simulink model "fmincon_in_simulink"  (R2022a)
settings: Solver=VariableStepAuto  StartTime=0.0  StopTime=10.0  RelTol=1e-3
libraries: slpidlib x8
settings Model: Creator=luca9  LastModifiedBy=luca9

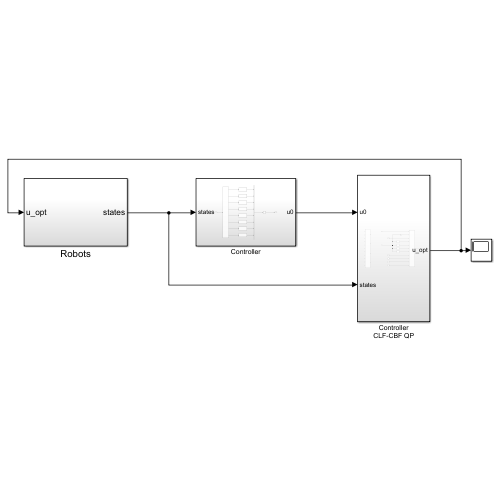
[thumbnail: Simulink's stored preview of the top-level diagram]
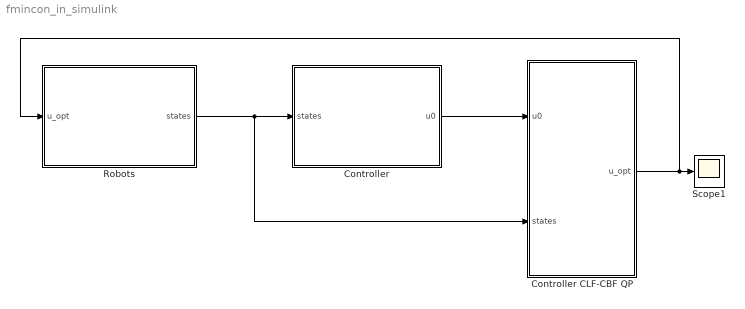
== system fmincon_in_simulink ==
  Controller : Subsystem
  Controller CLF-CBF QP : Subsystem
  Robots : Subsystem
  Scope1 : Scope
  wires:
  Controller CLF-CBF QP/1(u_opt) -> Robots/1(u_opt), Scope1/1
  Robots/1(states) -> Controller/1(states), Controller CLF-CBF QP/2(states)
  Controller/1(u0) -> Controller CLF-CBF QP/1(u0)

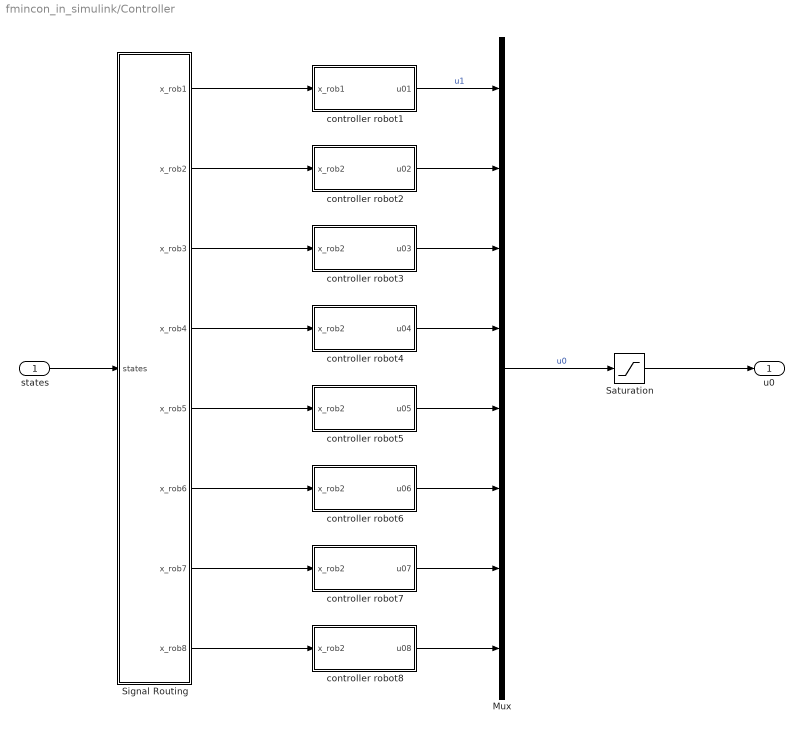
== system fmincon_in_simulink/Controller ==
  states : Inport
  Mux : Mux  Inputs=8
  Saturation : Saturate  UpperLimit=10  LowerLimit=-10
  Signal Routing : MATLAB Function  TreatAsAtomicUnit=on
  controller robot1 : Subsystem
  controller robot2 : Subsystem
  controller robot3 : Subsystem
  controller robot4 : Subsystem
  controller robot5 : Subsystem
  controller robot6 : Subsystem
  controller robot7 : Subsystem
  controller robot8 : Subsystem
  u0 : Outport
  wires:
  states/1 -> Signal Routing/1(states)
  Signal Routing/1(x_rob1) -> controller robot1/1(x_rob1)
  Signal Routing/2(x_rob2) -> controller robot2/1(x_rob2)
  Signal Routing/3(x_rob3) -> controller robot3/1(x_rob2)
  Signal Routing/4(x_rob4) -> controller robot4/1(x_rob2)
  Signal Routing/5(x_rob5) -> controller robot5/1(x_rob2)
  Signal Routing/6(x_rob6) -> controller robot6/1(x_rob2)
  Signal Routing/7(x_rob7) -> controller robot7/1(x_rob2)
  Signal Routing/8(x_rob8) -> controller robot8/1(x_rob2)
  controller robot1/1(u01) -> Mux/1  "u1"
  controller robot2/1(u02) -> Mux/2
  controller robot3/1(u03) -> Mux/3
  controller robot4/1(u04) -> Mux/4
  controller robot5/1(u05) -> Mux/5
  controller robot6/1(u06) -> Mux/6
  controller robot7/1(u07) -> Mux/7
  controller robot8/1(u08) -> Mux/8
  Mux/1 -> Saturation/1  "u0"
  Saturation/1 -> u0/1

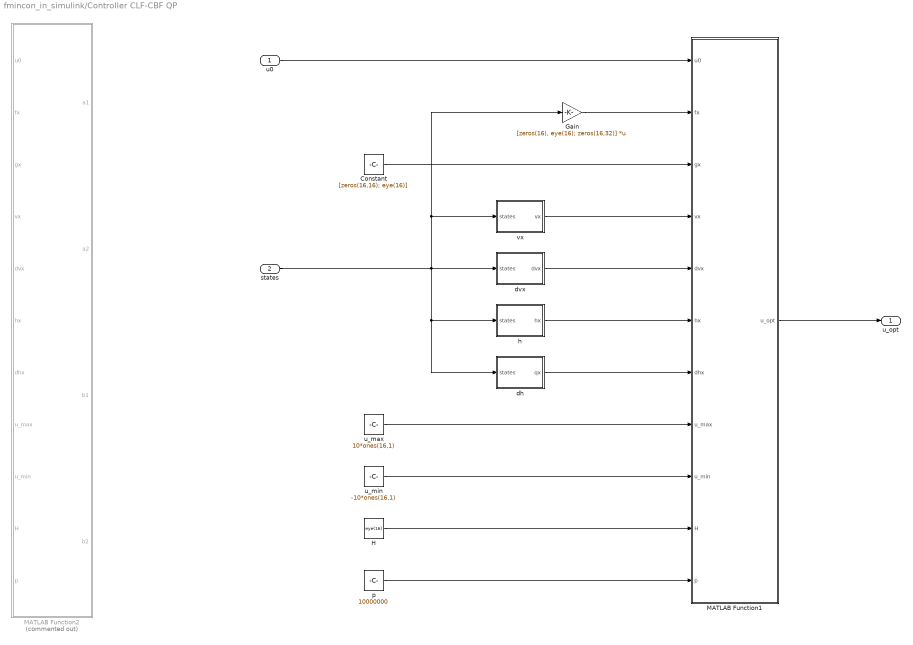
== system fmincon_in_simulink/Controller CLF-CBF QP ==
  u0 : Inport
  states : Inport  Port=2
  Constant : Constant  Value=[zeros(16,16); eye(16)]
  Gain : Gain  Gain=[zeros(16), eye(16); zeros(16,32)]  Multiplication=Matrix(K*u)
  H : Constant  Value=eye(16)
  MATLAB Function1 : MATLAB Function  TreatAsAtomicUnit=on
  MATLAB Function2 : MATLAB Function  Commented=on  TreatAsAtomicUnit=on
  dh : MATLAB Function  TreatAsAtomicUnit=on
  dvx : MATLAB Function  TreatAsAtomicUnit=on
  h : MATLAB Function  TreatAsAtomicUnit=on
  p : Constant  Value=10000000
  u_max : Constant  Value=10*ones(16,1)
  u_min : Constant  Value=-10*ones(16,1)
  vx : MATLAB Function  TreatAsAtomicUnit=on
  u_opt : Outport
  wires:
  u_min/1 -> MATLAB Function1/9(u_min)
  Gain/1 -> MATLAB Function1/2(fx)
  states/1 -> dh/1(states), h/1(states), Gain/1, vx/1(states), dvx/1(states)
  u_max/1 -> MATLAB Function1/8(u_max)
  Constant/1 -> MATLAB Function1/3(gx)
  h/1(hx) -> MATLAB Function1/6(hx)
  dh/1(qx) -> MATLAB Function1/7(dhx)
  H/1 -> MATLAB Function1/10(H)
  vx/1(vx) -> MATLAB Function1/4(vx)
  dvx/1(dvx) -> MATLAB Function1/5(dvx)
  p/1 -> MATLAB Function1/11(p)
  u0/1 -> MATLAB Function1/1(u0)
  MATLAB Function1/1(u_opt) -> u_opt/1

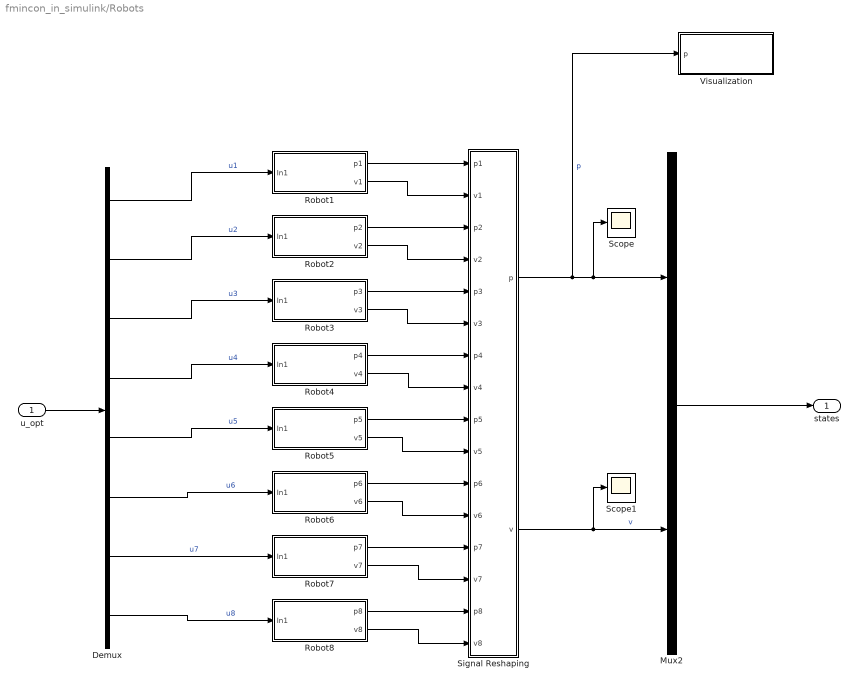
== system fmincon_in_simulink/Robots ==
  u_opt : Inport
  Demux : Demux  Outputs=8
  Mux2 : Mux  Inputs=2
  Robot1 : Subsystem
  Robot2 : Subsystem
  Robot3 : Subsystem
  Robot4 : Subsystem
  Robot5 : Subsystem
  Robot6 : Subsystem
  Robot7 : Subsystem
  Robot8 : Subsystem
  Scope : Scope
  Scope1 : Scope
  Signal Reshaping : MATLAB Function  TreatAsAtomicUnit=on
  Visualization : Subsystem
  states : Outport
  wires:
  u_opt/1 -> Demux/1
  Demux/1 -> Robot1/1(In1)  "u1"
  Demux/2 -> Robot2/1(In1)  "u2"
  Demux/3 -> Robot3/1(In1)  "u3"
  Demux/4 -> Robot4/1(In1)  "u4"
  Demux/5 -> Robot5/1(In1)  "u5"
  Demux/6 -> Robot6/1(In1)  "u6"
  Demux/7 -> Robot7/1(In1)  "u7"
  Demux/8 -> Robot8/1(In1)  "u8"
  Mux2/1 -> states/1
  Signal Reshaping/2(v) -> Scope1/1, Mux2/2  "v"
  Signal Reshaping/1(p) -> Visualization/1(p), Scope/1, Mux2/1  "p"
  Robot1/1(p1) -> Signal Reshaping/1(p1)
  Robot1/2(v1) -> Signal Reshaping/2(v1)
  Robot2/1(p2) -> Signal Reshaping/3(p2)
  Robot2/2(v2) -> Signal Reshaping/4(v2)
  Robot3/1(p3) -> Signal Reshaping/5(p3)
  Robot3/2(v3) -> Signal Reshaping/6(v3)
  Robot4/1(p4) -> Signal Reshaping/7(p4)
  Robot4/2(v4) -> Signal Reshaping/8(v4)
  Robot5/1(p5) -> Signal Reshaping/9(p5)
  Robot5/2(v5) -> Signal Reshaping/10(v5)
  Robot6/1(p6) -> Signal Reshaping/11(p6)
  Robot6/2(v6) -> Signal Reshaping/12(v6)
  Robot7/1(p7) -> Signal Reshaping/13(p7)
  Robot7/2(v7) -> Signal Reshaping/14(v7)
  Robot8/1(p8) -> Signal Reshaping/15(p8)
  Robot8/2(v8) -> Signal Reshaping/16(v8)

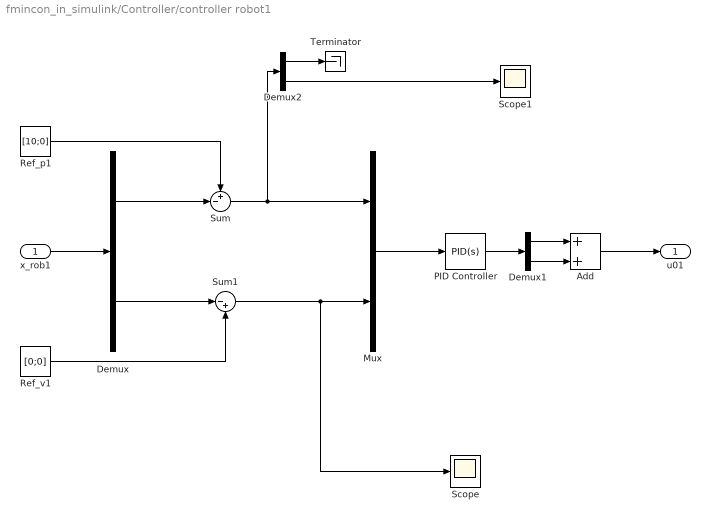
== system fmincon_in_simulink/Controller/controller robot1 ==
  x_rob1 : Inport
  Add : Sum
  Demux : Demux  Outputs=2
  Demux1 : Demux  Outputs=2
  Demux2 : Demux  Outputs=2
  Mux : Mux  Inputs=2
  PID Controller : slpidlib/PID Controller  Controller=PID  Form=Parallel  TimeDomain=Continuous-time  UseExternalTs=off  SampleTime=-1  IntegratorMethod=Forward Euler  FilterMethod=Forward Euler  ControllerParametersSource=internal  P=5  I=0.0000001  UseKiTs=off  D=0.01  N=1  UseFilter=on  TunerSelectOption=Transfer Function Based (PID Tuner App)  InitialConditionSource=internal  InitialConditionForIntegrator=0  InitialConditionForFilter=0  DifferentiatorICPrevScaledInput=0  ExternalReset=none  TrackingMode=off  Kt=1  LimitOutput=off  SatLimitsSource=internal  UpperSaturationLimit=inf  LowerSaturationLimit=-inf  LinearizeAsGain=on  AntiWindupMode=none  Kb=1  POutMin=[]  POutMax=[]  IOutMin=[]  IOutMax=[]  DOutMin=[]  DOutMax=[]  NOutMin=[]  NOutMax=[]  SumOutMin=[]  SumOutMax=[]  SaturationOutMin=[]  SaturationOutMax=[]  PParamMin=[]  PParamMax=[]  IParamMin=[]  IParamMax=[]  DParamMin=[]  DParamMax=[]  NParamMin=[]  NParamMax=[]  KbParamMin=[]  KbParamMax=[]  KtParamMin=[]  KtParamMax=[]  KbOutMin=[]  KbOutMax=[]  KtOutMin=[]  KtOutMax=[]  IntegratorOutMin=[]  IntegratorOutMax=[]  FilterOutMin=[]  FilterOutMax=[]  SumI1OutMin=[]  SumI1OutMax=[]  SumI2OutMin=[]  SumI2OutMax=[]  SumI3OutMin=[]  SumI3OutMax=[]  SumI4OutMin=[]  SumI4OutMax=[]  SumDOutMin=[]  SumDOutMax=[]  DifferentiatorOutMin=[]  DifferentiatorOutMax=[]  FilterDiffOutCoefMin=[]  FilterDiffOutCoefMax=[]  ReciprocalOutMin=[]  ReciprocalOutMax=[]  SumDenOutMin=[]  SumDenOutMax=[]  SumNumOutMin=[]  SumNumOutMax=[]  DivideOutMin=[]  DivideOutMax=[]  UdiffTsProdOutMin=[]  UdiffTsProdOutMax=[]  NTsProdOutMin=[]  NTsProdOutMax=[]  UintegralTsProdOutMin=[]  UintegralTsProdOutMax=[]  UngainTsProdOutMin=[]  UngainTsProdOutMax=[]  IntegratorContinuousStateAttributes=''  IntegratorStateMustResolveToSignalObject=off  IntegratorRTWStateStorageClass=Auto  FilterContinuousStateAttributes=''  FilterStateMustResolveToSignalObject=off  FilterRTWStateStorageClass=Auto  ParallelPVariant=InternalParameters  IdealPVariant=Disabled  IVariant=InternalParameters  DVariant=InternalParameters  IntegratorVariant=Continuous  SatVariant=Disabled  AWVariant=Passthrough  PCopyVariant=Disabled  TRVariant=Disabled  FdbkBlocksVariant=Forward  IdealPFdbkVariant=Disabled  SatFdbkVariant=Disabled  DerivativeFilterVariant=ContFilter  NVariant=InternalParameters  NCopyVariant=Disabled  FilterICVariant=InternalICsFilter  IntegratorICVariant=InternalICs  ExternalResetVariant=Disabled  TRSumVariant=Passthrough  SumFdbkVariant=Disabled  SumVariant=Sum_PID  TsampFilterVariant=InternalTs  TsampNgainVariant=Passthrough  TsampIntegralVariant=Passthrough  ExternalSaturationOutDataTypeStr=Inherit: Same as second input  aMode=0
  Ref_p1 : Constant  Value=[10;0]  VectorParams1D=off
  Ref_v1 : Constant  Value=[0;0]  VectorParams1D=off
  Scope : Scope
  Scope1 : Scope
  Sum : Sum  Inputs=+-|
  Sum1 : Sum  Inputs=|-+
  Terminator : Terminator
  u01 : Outport
  wires:
  x_rob1/1 -> Demux/1
  Demux/1 -> Sum/2
  Ref_p1/1 -> Sum/1
  Demux/2 -> Sum1/1
  Ref_v1/1 -> Sum1/2
  Sum/1 -> Mux/1, Demux2/1
  Sum1/1 -> Mux/2, Scope/1
  Mux/1 -> PID Controller/1
  PID Controller/1 -> Demux1/1
  Demux1/2 -> Add/2
  Demux1/1 -> Add/1
  Add/1 -> u01/1
  Demux2/1 -> Terminator/1
  Demux2/2 -> Scope1/1

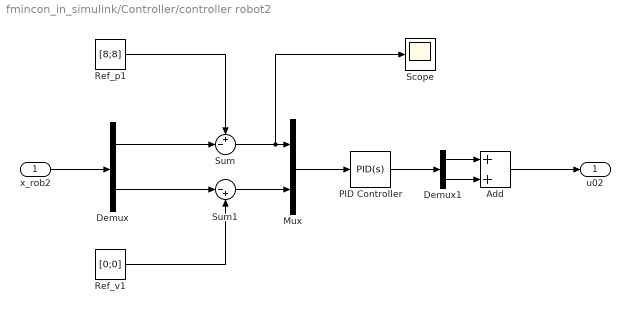
== system fmincon_in_simulink/Controller/controller robot2 ==
  x_rob2 : Inport
  Add : Sum
  Demux : Demux  Outputs=2
  Demux1 : Demux  Outputs=2
  Mux : Mux  Inputs=2
  PID Controller : slpidlib/PID Controller  Controller=PID  Form=Parallel  TimeDomain=Continuous-time  UseExternalTs=off  SampleTime=-1  IntegratorMethod=Forward Euler  FilterMethod=Forward Euler  ControllerParametersSource=internal  P=5  I=0.0000001  UseKiTs=off  D=0.01  N=1  UseFilter=on  TunerSelectOption=Transfer Function Based (PID Tuner App)  InitialConditionSource=internal  InitialConditionForIntegrator=0  InitialConditionForFilter=0  DifferentiatorICPrevScaledInput=0  ExternalReset=none  TrackingMode=off  Kt=1  LimitOutput=off  SatLimitsSource=internal  UpperSaturationLimit=inf  LowerSaturationLimit=-inf  LinearizeAsGain=on  AntiWindupMode=none  Kb=1  POutMin=[]  POutMax=[]  IOutMin=[]  IOutMax=[]  DOutMin=[]  DOutMax=[]  NOutMin=[]  NOutMax=[]  SumOutMin=[]  SumOutMax=[]  SaturationOutMin=[]  SaturationOutMax=[]  PParamMin=[]  PParamMax=[]  IParamMin=[]  IParamMax=[]  DParamMin=[]  DParamMax=[]  NParamMin=[]  NParamMax=[]  KbParamMin=[]  KbParamMax=[]  KtParamMin=[]  KtParamMax=[]  KbOutMin=[]  KbOutMax=[]  KtOutMin=[]  KtOutMax=[]  IntegratorOutMin=[]  IntegratorOutMax=[]  FilterOutMin=[]  FilterOutMax=[]  SumI1OutMin=[]  SumI1OutMax=[]  SumI2OutMin=[]  SumI2OutMax=[]  SumI3OutMin=[]  SumI3OutMax=[]  SumI4OutMin=[]  SumI4OutMax=[]  SumDOutMin=[]  SumDOutMax=[]  DifferentiatorOutMin=[]  DifferentiatorOutMax=[]  FilterDiffOutCoefMin=[]  FilterDiffOutCoefMax=[]  ReciprocalOutMin=[]  ReciprocalOutMax=[]  SumDenOutMin=[]  SumDenOutMax=[]  SumNumOutMin=[]  SumNumOutMax=[]  DivideOutMin=[]  DivideOutMax=[]  UdiffTsProdOutMin=[]  UdiffTsProdOutMax=[]  NTsProdOutMin=[]  NTsProdOutMax=[]  UintegralTsProdOutMin=[]  UintegralTsProdOutMax=[]  UngainTsProdOutMin=[]  UngainTsProdOutMax=[]  IntegratorContinuousStateAttributes=''  IntegratorStateMustResolveToSignalObject=off  IntegratorRTWStateStorageClass=Auto  FilterContinuousStateAttributes=''  FilterStateMustResolveToSignalObject=off  FilterRTWStateStorageClass=Auto  ParallelPVariant=InternalParameters  IdealPVariant=Disabled  IVariant=InternalParameters  DVariant=InternalParameters  IntegratorVariant=Continuous  SatVariant=Disabled  AWVariant=Passthrough  PCopyVariant=Disabled  TRVariant=Disabled  FdbkBlocksVariant=Forward  IdealPFdbkVariant=Disabled  SatFdbkVariant=Disabled  DerivativeFilterVariant=ContFilter  NVariant=InternalParameters  NCopyVariant=Disabled  FilterICVariant=InternalICsFilter  IntegratorICVariant=InternalICs  ExternalResetVariant=Disabled  TRSumVariant=Passthrough  SumFdbkVariant=Disabled  SumVariant=Sum_PID  TsampFilterVariant=InternalTs  TsampNgainVariant=Passthrough  TsampIntegralVariant=Passthrough  ExternalSaturationOutDataTypeStr=Inherit: Same as second input  aMode=0
  Ref_p1 : Constant  Value=[8;8]  VectorParams1D=off
  Ref_v1 : Constant  Value=[0;0]  VectorParams1D=off
  Scope : Scope
  Sum : Sum  Inputs=+-|
  Sum1 : Sum  Inputs=|-+
  u02 : Outport
  wires:
  x_rob2/1 -> Demux/1
  Demux/1 -> Sum/2
  Ref_p1/1 -> Sum/1
  Demux/2 -> Sum1/1
  Ref_v1/1 -> Sum1/2
  Add/1 -> u02/1
  Demux1/2 -> Add/2
  Mux/1 -> PID Controller/1
  Sum/1 -> Scope/1, Mux/1
  Sum1/1 -> Mux/2
  PID Controller/1 -> Demux1/1
  Demux1/1 -> Add/1

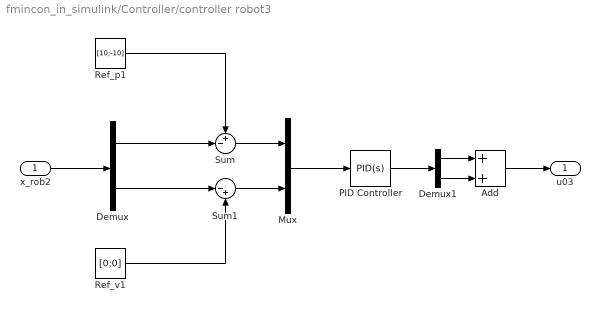
== system fmincon_in_simulink/Controller/controller robot3 ==
  x_rob2 : Inport
  Add : Sum
  Demux : Demux  Outputs=2
  Demux1 : Demux  Outputs=2
  Mux : Mux  Inputs=2
  PID Controller : slpidlib/PID Controller  Controller=PID  Form=Parallel  TimeDomain=Continuous-time  UseExternalTs=off  SampleTime=-1  IntegratorMethod=Forward Euler  FilterMethod=Forward Euler  ControllerParametersSource=internal  P=5  I=0.0000001  UseKiTs=off  D=0.01  N=1  UseFilter=on  TunerSelectOption=Transfer Function Based (PID Tuner App)  InitialConditionSource=internal  InitialConditionForIntegrator=0  InitialConditionForFilter=0  DifferentiatorICPrevScaledInput=0  ExternalReset=none  TrackingMode=off  Kt=1  LimitOutput=off  SatLimitsSource=internal  UpperSaturationLimit=inf  LowerSaturationLimit=-inf  LinearizeAsGain=on  AntiWindupMode=none  Kb=1  POutMin=[]  POutMax=[]  IOutMin=[]  IOutMax=[]  DOutMin=[]  DOutMax=[]  NOutMin=[]  NOutMax=[]  SumOutMin=[]  SumOutMax=[]  SaturationOutMin=[]  SaturationOutMax=[]  PParamMin=[]  PParamMax=[]  IParamMin=[]  IParamMax=[]  DParamMin=[]  DParamMax=[]  NParamMin=[]  NParamMax=[]  KbParamMin=[]  KbParamMax=[]  KtParamMin=[]  KtParamMax=[]  KbOutMin=[]  KbOutMax=[]  KtOutMin=[]  KtOutMax=[]  IntegratorOutMin=[]  IntegratorOutMax=[]  FilterOutMin=[]  FilterOutMax=[]  SumI1OutMin=[]  SumI1OutMax=[]  SumI2OutMin=[]  SumI2OutMax=[]  SumI3OutMin=[]  SumI3OutMax=[]  SumI4OutMin=[]  SumI4OutMax=[]  SumDOutMin=[]  SumDOutMax=[]  DifferentiatorOutMin=[]  DifferentiatorOutMax=[]  FilterDiffOutCoefMin=[]  FilterDiffOutCoefMax=[]  ReciprocalOutMin=[]  ReciprocalOutMax=[]  SumDenOutMin=[]  SumDenOutMax=[]  SumNumOutMin=[]  SumNumOutMax=[]  DivideOutMin=[]  DivideOutMax=[]  UdiffTsProdOutMin=[]  UdiffTsProdOutMax=[]  NTsProdOutMin=[]  NTsProdOutMax=[]  UintegralTsProdOutMin=[]  UintegralTsProdOutMax=[]  UngainTsProdOutMin=[]  UngainTsProdOutMax=[]  IntegratorContinuousStateAttributes=''  IntegratorStateMustResolveToSignalObject=off  IntegratorRTWStateStorageClass=Auto  FilterContinuousStateAttributes=''  FilterStateMustResolveToSignalObject=off  FilterRTWStateStorageClass=Auto  ParallelPVariant=InternalParameters  IdealPVariant=Disabled  IVariant=InternalParameters  DVariant=InternalParameters  IntegratorVariant=Continuous  SatVariant=Disabled  AWVariant=Passthrough  PCopyVariant=Disabled  TRVariant=Disabled  FdbkBlocksVariant=Forward  IdealPFdbkVariant=Disabled  SatFdbkVariant=Disabled  DerivativeFilterVariant=ContFilter  NVariant=InternalParameters  NCopyVariant=Disabled  FilterICVariant=InternalICsFilter  IntegratorICVariant=InternalICs  ExternalResetVariant=Disabled  TRSumVariant=Passthrough  SumFdbkVariant=Disabled  SumVariant=Sum_PID  TsampFilterVariant=InternalTs  TsampNgainVariant=Passthrough  TsampIntegralVariant=Passthrough  ExternalSaturationOutDataTypeStr=Inherit: Same as second input  aMode=0
  Ref_p1 : Constant  Value=[10;-10]  VectorParams1D=off
  Ref_v1 : Constant  Value=[0;0]  VectorParams1D=off
  Sum : Sum  Inputs=+-|
  Sum1 : Sum  Inputs=|-+
  u03 : Outport
  wires:
  x_rob2/1 -> Demux/1
  Demux/1 -> Sum/2
  Ref_p1/1 -> Sum/1
  Demux/2 -> Sum1/1
  Ref_v1/1 -> Sum1/2
  Add/1 -> u03/1
  Demux1/2 -> Add/2
  Demux1/1 -> Add/1
  Sum1/1 -> Mux/2
  Sum/1 -> Mux/1
  PID Controller/1 -> Demux1/1
  Mux/1 -> PID Controller/1

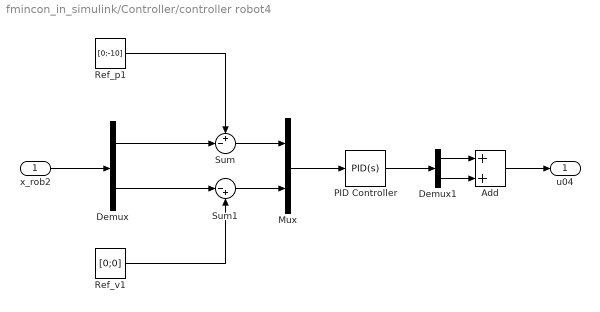
== system fmincon_in_simulink/Controller/controller robot4 ==
  x_rob2 : Inport
  Add : Sum
  Demux : Demux  Outputs=2
  Demux1 : Demux  Outputs=2
  Mux : Mux  Inputs=2
  PID Controller : slpidlib/PID Controller  Controller=PID  Form=Parallel  TimeDomain=Continuous-time  UseExternalTs=off  SampleTime=-1  IntegratorMethod=Forward Euler  FilterMethod=Forward Euler  ControllerParametersSource=internal  P=5  I=0.0000001  UseKiTs=off  D=0.01  N=1  UseFilter=on  TunerSelectOption=Transfer Function Based (PID Tuner App)  InitialConditionSource=internal  InitialConditionForIntegrator=0  InitialConditionForFilter=0  DifferentiatorICPrevScaledInput=0  ExternalReset=none  TrackingMode=off  Kt=1  LimitOutput=off  SatLimitsSource=internal  UpperSaturationLimit=inf  LowerSaturationLimit=-inf  LinearizeAsGain=on  AntiWindupMode=none  Kb=1  POutMin=[]  POutMax=[]  IOutMin=[]  IOutMax=[]  DOutMin=[]  DOutMax=[]  NOutMin=[]  NOutMax=[]  SumOutMin=[]  SumOutMax=[]  SaturationOutMin=[]  SaturationOutMax=[]  PParamMin=[]  PParamMax=[]  IParamMin=[]  IParamMax=[]  DParamMin=[]  DParamMax=[]  NParamMin=[]  NParamMax=[]  KbParamMin=[]  KbParamMax=[]  KtParamMin=[]  KtParamMax=[]  KbOutMin=[]  KbOutMax=[]  KtOutMin=[]  KtOutMax=[]  IntegratorOutMin=[]  IntegratorOutMax=[]  FilterOutMin=[]  FilterOutMax=[]  SumI1OutMin=[]  SumI1OutMax=[]  SumI2OutMin=[]  SumI2OutMax=[]  SumI3OutMin=[]  SumI3OutMax=[]  SumI4OutMin=[]  SumI4OutMax=[]  SumDOutMin=[]  SumDOutMax=[]  DifferentiatorOutMin=[]  DifferentiatorOutMax=[]  FilterDiffOutCoefMin=[]  FilterDiffOutCoefMax=[]  ReciprocalOutMin=[]  ReciprocalOutMax=[]  SumDenOutMin=[]  SumDenOutMax=[]  SumNumOutMin=[]  SumNumOutMax=[]  DivideOutMin=[]  DivideOutMax=[]  UdiffTsProdOutMin=[]  UdiffTsProdOutMax=[]  NTsProdOutMin=[]  NTsProdOutMax=[]  UintegralTsProdOutMin=[]  UintegralTsProdOutMax=[]  UngainTsProdOutMin=[]  UngainTsProdOutMax=[]  IntegratorContinuousStateAttributes=''  IntegratorStateMustResolveToSignalObject=off  IntegratorRTWStateStorageClass=Auto  FilterContinuousStateAttributes=''  FilterStateMustResolveToSignalObject=off  FilterRTWStateStorageClass=Auto  ParallelPVariant=InternalParameters  IdealPVariant=Disabled  IVariant=InternalParameters  DVariant=InternalParameters  IntegratorVariant=Continuous  SatVariant=Disabled  AWVariant=Passthrough  PCopyVariant=Disabled  TRVariant=Disabled  FdbkBlocksVariant=Forward  IdealPFdbkVariant=Disabled  SatFdbkVariant=Disabled  DerivativeFilterVariant=ContFilter  NVariant=InternalParameters  NCopyVariant=Disabled  FilterICVariant=InternalICsFilter  IntegratorICVariant=InternalICs  ExternalResetVariant=Disabled  TRSumVariant=Passthrough  SumFdbkVariant=Disabled  SumVariant=Sum_PID  TsampFilterVariant=InternalTs  TsampNgainVariant=Passthrough  TsampIntegralVariant=Passthrough  ExternalSaturationOutDataTypeStr=Inherit: Same as second input  aMode=0
  Ref_p1 : Constant  Value=[0;-10]  VectorParams1D=off
  Ref_v1 : Constant  Value=[0;0]  VectorParams1D=off
  Sum : Sum  Inputs=+-|
  Sum1 : Sum  Inputs=|-+
  u04 : Outport
  wires:
  x_rob2/1 -> Demux/1
  Demux/1 -> Sum/2
  Ref_p1/1 -> Sum/1
  Demux/2 -> Sum1/1
  Ref_v1/1 -> Sum1/2
  PID Controller/1 -> Demux1/1
  Demux1/2 -> Add/2
  Add/1 -> u04/1
  Demux1/1 -> Add/1
  Mux/1 -> PID Controller/1
  Sum1/1 -> Mux/2
  Sum/1 -> Mux/1

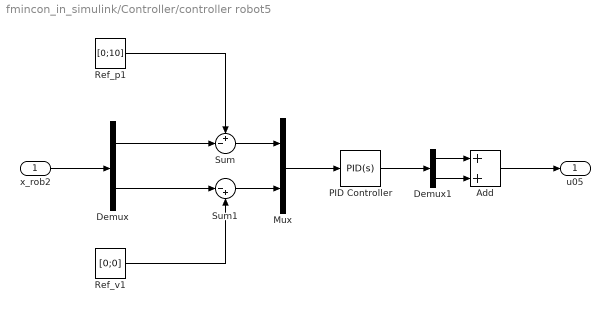
== system fmincon_in_simulink/Controller/controller robot5 ==
  x_rob2 : Inport
  Add : Sum
  Demux : Demux  Outputs=2
  Demux1 : Demux  Outputs=2
  Mux : Mux  Inputs=2
  PID Controller : slpidlib/PID Controller  Controller=PID  Form=Parallel  TimeDomain=Continuous-time  UseExternalTs=off  SampleTime=-1  IntegratorMethod=Forward Euler  FilterMethod=Forward Euler  ControllerParametersSource=internal  P=5  I=0  UseKiTs=off  D=0  N=100  UseFilter=on  TunerSelectOption=Transfer Function Based (PID Tuner App)  InitialConditionSource=internal  InitialConditionForIntegrator=0  InitialConditionForFilter=0  DifferentiatorICPrevScaledInput=0  ExternalReset=none  TrackingMode=off  Kt=1  LimitOutput=off  SatLimitsSource=internal  UpperSaturationLimit=inf  LowerSaturationLimit=-inf  LinearizeAsGain=on  AntiWindupMode=none  Kb=1  POutMin=[]  POutMax=[]  IOutMin=[]  IOutMax=[]  DOutMin=[]  DOutMax=[]  NOutMin=[]  NOutMax=[]  SumOutMin=[]  SumOutMax=[]  SaturationOutMin=[]  SaturationOutMax=[]  PParamMin=[]  PParamMax=[]  IParamMin=[]  IParamMax=[]  DParamMin=[]  DParamMax=[]  NParamMin=[]  NParamMax=[]  KbParamMin=[]  KbParamMax=[]  KtParamMin=[]  KtParamMax=[]  KbOutMin=[]  KbOutMax=[]  KtOutMin=[]  KtOutMax=[]  IntegratorOutMin=[]  IntegratorOutMax=[]  FilterOutMin=[]  FilterOutMax=[]  SumI1OutMin=[]  SumI1OutMax=[]  SumI2OutMin=[]  SumI2OutMax=[]  SumI3OutMin=[]  SumI3OutMax=[]  SumI4OutMin=[]  SumI4OutMax=[]  SumDOutMin=[]  SumDOutMax=[]  DifferentiatorOutMin=[]  DifferentiatorOutMax=[]  FilterDiffOutCoefMin=[]  FilterDiffOutCoefMax=[]  ReciprocalOutMin=[]  ReciprocalOutMax=[]  SumDenOutMin=[]  SumDenOutMax=[]  SumNumOutMin=[]  SumNumOutMax=[]  DivideOutMin=[]  DivideOutMax=[]  UdiffTsProdOutMin=[]  UdiffTsProdOutMax=[]  NTsProdOutMin=[]  NTsProdOutMax=[]  UintegralTsProdOutMin=[]  UintegralTsProdOutMax=[]  UngainTsProdOutMin=[]  UngainTsProdOutMax=[]  IntegratorContinuousStateAttributes=''  IntegratorStateMustResolveToSignalObject=off  IntegratorRTWStateStorageClass=Auto  FilterContinuousStateAttributes=''  FilterStateMustResolveToSignalObject=off  FilterRTWStateStorageClass=Auto  ParallelPVariant=InternalParameters  IdealPVariant=Disabled  IVariant=InternalParameters  DVariant=InternalParameters  IntegratorVariant=Continuous  SatVariant=Disabled  AWVariant=Passthrough  PCopyVariant=Disabled  TRVariant=Disabled  FdbkBlocksVariant=Forward  IdealPFdbkVariant=Disabled  SatFdbkVariant=Disabled  DerivativeFilterVariant=ContFilter  NVariant=InternalParameters  NCopyVariant=Disabled  FilterICVariant=InternalICsFilter  IntegratorICVariant=InternalICs  ExternalResetVariant=Disabled  TRSumVariant=Passthrough  SumFdbkVariant=Disabled  SumVariant=Sum_PID  TsampFilterVariant=InternalTs  TsampNgainVariant=Passthrough  TsampIntegralVariant=Passthrough  ExternalSaturationOutDataTypeStr=Inherit: Same as second input  aMode=0
  Ref_p1 : Constant  Value=[0;10]  VectorParams1D=off
  Ref_v1 : Constant  Value=[0;0]  VectorParams1D=off
  Sum : Sum  Inputs=+-|
  Sum1 : Sum  Inputs=|-+
  u05 : Outport
  wires:
  x_rob2/1 -> Demux/1
  Demux/1 -> Sum/2
  Ref_p1/1 -> Sum/1
  Demux/2 -> Sum1/1
  Ref_v1/1 -> Sum1/2
  Add/1 -> u05/1
  PID Controller/1 -> Demux1/1
  Demux1/2 -> Add/2
  Demux1/1 -> Add/1
  Mux/1 -> PID Controller/1
  Sum1/1 -> Mux/2
  Sum/1 -> Mux/1

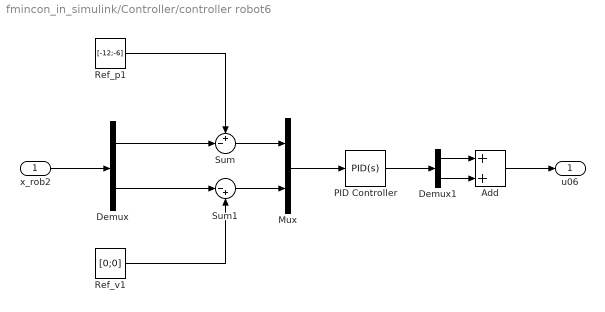
== system fmincon_in_simulink/Controller/controller robot6 ==
  x_rob2 : Inport
  Add : Sum
  Demux : Demux  Outputs=2
  Demux1 : Demux  Outputs=2
  Mux : Mux  Inputs=2
  PID Controller : slpidlib/PID Controller  Controller=PID  Form=Parallel  TimeDomain=Continuous-time  UseExternalTs=off  SampleTime=-1  IntegratorMethod=Forward Euler  FilterMethod=Forward Euler  ControllerParametersSource=internal  P=5  I=0  UseKiTs=off  D=0  N=100  UseFilter=on  TunerSelectOption=Transfer Function Based (PID Tuner App)  InitialConditionSource=internal  InitialConditionForIntegrator=0  InitialConditionForFilter=0  DifferentiatorICPrevScaledInput=0  ExternalReset=none  TrackingMode=off  Kt=1  LimitOutput=off  SatLimitsSource=internal  UpperSaturationLimit=inf  LowerSaturationLimit=-inf  LinearizeAsGain=on  AntiWindupMode=none  Kb=1  POutMin=[]  POutMax=[]  IOutMin=[]  IOutMax=[]  DOutMin=[]  DOutMax=[]  NOutMin=[]  NOutMax=[]  SumOutMin=[]  SumOutMax=[]  SaturationOutMin=[]  SaturationOutMax=[]  PParamMin=[]  PParamMax=[]  IParamMin=[]  IParamMax=[]  DParamMin=[]  DParamMax=[]  NParamMin=[]  NParamMax=[]  KbParamMin=[]  KbParamMax=[]  KtParamMin=[]  KtParamMax=[]  KbOutMin=[]  KbOutMax=[]  KtOutMin=[]  KtOutMax=[]  IntegratorOutMin=[]  IntegratorOutMax=[]  FilterOutMin=[]  FilterOutMax=[]  SumI1OutMin=[]  SumI1OutMax=[]  SumI2OutMin=[]  SumI2OutMax=[]  SumI3OutMin=[]  SumI3OutMax=[]  SumI4OutMin=[]  SumI4OutMax=[]  SumDOutMin=[]  SumDOutMax=[]  DifferentiatorOutMin=[]  DifferentiatorOutMax=[]  FilterDiffOutCoefMin=[]  FilterDiffOutCoefMax=[]  ReciprocalOutMin=[]  ReciprocalOutMax=[]  SumDenOutMin=[]  SumDenOutMax=[]  SumNumOutMin=[]  SumNumOutMax=[]  DivideOutMin=[]  DivideOutMax=[]  UdiffTsProdOutMin=[]  UdiffTsProdOutMax=[]  NTsProdOutMin=[]  NTsProdOutMax=[]  UintegralTsProdOutMin=[]  UintegralTsProdOutMax=[]  UngainTsProdOutMin=[]  UngainTsProdOutMax=[]  IntegratorContinuousStateAttributes=''  IntegratorStateMustResolveToSignalObject=off  IntegratorRTWStateStorageClass=Auto  FilterContinuousStateAttributes=''  FilterStateMustResolveToSignalObject=off  FilterRTWStateStorageClass=Auto  ParallelPVariant=InternalParameters  IdealPVariant=Disabled  IVariant=InternalParameters  DVariant=InternalParameters  IntegratorVariant=Continuous  SatVariant=Disabled  AWVariant=Passthrough  PCopyVariant=Disabled  TRVariant=Disabled  FdbkBlocksVariant=Forward  IdealPFdbkVariant=Disabled  SatFdbkVariant=Disabled  DerivativeFilterVariant=ContFilter  NVariant=InternalParameters  NCopyVariant=Disabled  FilterICVariant=InternalICsFilter  IntegratorICVariant=InternalICs  ExternalResetVariant=Disabled  TRSumVariant=Passthrough  SumFdbkVariant=Disabled  SumVariant=Sum_PID  TsampFilterVariant=InternalTs  TsampNgainVariant=Passthrough  TsampIntegralVariant=Passthrough  ExternalSaturationOutDataTypeStr=Inherit: Same as second input  aMode=0
  Ref_p1 : Constant  Value=[-12;-6]  VectorParams1D=off
  Ref_v1 : Constant  Value=[0;0]  VectorParams1D=off
  Sum : Sum  Inputs=+-|
  Sum1 : Sum  Inputs=|-+
  u06 : Outport
  wires:
  x_rob2/1 -> Demux/1
  Demux/1 -> Sum/2
  Ref_p1/1 -> Sum/1
  Demux/2 -> Sum1/1
  Ref_v1/1 -> Sum1/2
  PID Controller/1 -> Demux1/1
  Demux1/2 -> Add/2
  Add/1 -> u06/1
  Demux1/1 -> Add/1
  Mux/1 -> PID Controller/1
  Sum1/1 -> Mux/2
  Sum/1 -> Mux/1

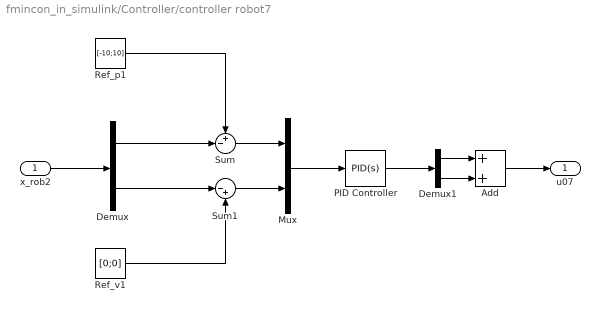
== system fmincon_in_simulink/Controller/controller robot7 ==
  x_rob2 : Inport
  Add : Sum
  Demux : Demux  Outputs=2
  Demux1 : Demux  Outputs=2
  Mux : Mux  Inputs=2
  PID Controller : slpidlib/PID Controller  Controller=PID  Form=Parallel  TimeDomain=Continuous-time  UseExternalTs=off  SampleTime=-1  IntegratorMethod=Forward Euler  FilterMethod=Forward Euler  ControllerParametersSource=internal  P=5  I=0  UseKiTs=off  D=0  N=100  UseFilter=on  TunerSelectOption=Transfer Function Based (PID Tuner App)  InitialConditionSource=internal  InitialConditionForIntegrator=0  InitialConditionForFilter=0  DifferentiatorICPrevScaledInput=0  ExternalReset=none  TrackingMode=off  Kt=1  LimitOutput=off  SatLimitsSource=internal  UpperSaturationLimit=inf  LowerSaturationLimit=-inf  LinearizeAsGain=on  AntiWindupMode=none  Kb=1  POutMin=[]  POutMax=[]  IOutMin=[]  IOutMax=[]  DOutMin=[]  DOutMax=[]  NOutMin=[]  NOutMax=[]  SumOutMin=[]  SumOutMax=[]  SaturationOutMin=[]  SaturationOutMax=[]  PParamMin=[]  PParamMax=[]  IParamMin=[]  IParamMax=[]  DParamMin=[]  DParamMax=[]  NParamMin=[]  NParamMax=[]  KbParamMin=[]  KbParamMax=[]  KtParamMin=[]  KtParamMax=[]  KbOutMin=[]  KbOutMax=[]  KtOutMin=[]  KtOutMax=[]  IntegratorOutMin=[]  IntegratorOutMax=[]  FilterOutMin=[]  FilterOutMax=[]  SumI1OutMin=[]  SumI1OutMax=[]  SumI2OutMin=[]  SumI2OutMax=[]  SumI3OutMin=[]  SumI3OutMax=[]  SumI4OutMin=[]  SumI4OutMax=[]  SumDOutMin=[]  SumDOutMax=[]  DifferentiatorOutMin=[]  DifferentiatorOutMax=[]  FilterDiffOutCoefMin=[]  FilterDiffOutCoefMax=[]  ReciprocalOutMin=[]  ReciprocalOutMax=[]  SumDenOutMin=[]  SumDenOutMax=[]  SumNumOutMin=[]  SumNumOutMax=[]  DivideOutMin=[]  DivideOutMax=[]  UdiffTsProdOutMin=[]  UdiffTsProdOutMax=[]  NTsProdOutMin=[]  NTsProdOutMax=[]  UintegralTsProdOutMin=[]  UintegralTsProdOutMax=[]  UngainTsProdOutMin=[]  UngainTsProdOutMax=[]  IntegratorContinuousStateAttributes=''  IntegratorStateMustResolveToSignalObject=off  IntegratorRTWStateStorageClass=Auto  FilterContinuousStateAttributes=''  FilterStateMustResolveToSignalObject=off  FilterRTWStateStorageClass=Auto  ParallelPVariant=InternalParameters  IdealPVariant=Disabled  IVariant=InternalParameters  DVariant=InternalParameters  IntegratorVariant=Continuous  SatVariant=Disabled  AWVariant=Passthrough  PCopyVariant=Disabled  TRVariant=Disabled  FdbkBlocksVariant=Forward  IdealPFdbkVariant=Disabled  SatFdbkVariant=Disabled  DerivativeFilterVariant=ContFilter  NVariant=InternalParameters  NCopyVariant=Disabled  FilterICVariant=InternalICsFilter  IntegratorICVariant=InternalICs  ExternalResetVariant=Disabled  TRSumVariant=Passthrough  SumFdbkVariant=Disabled  SumVariant=Sum_PID  TsampFilterVariant=InternalTs  TsampNgainVariant=Passthrough  TsampIntegralVariant=Passthrough  ExternalSaturationOutDataTypeStr=Inherit: Same as second input  aMode=0
  Ref_p1 : Constant  Value=[-10;10]  VectorParams1D=off
  Ref_v1 : Constant  Value=[0;0]  VectorParams1D=off
  Sum : Sum  Inputs=+-|
  Sum1 : Sum  Inputs=|-+
  u07 : Outport
  wires:
  x_rob2/1 -> Demux/1
  Demux/1 -> Sum/2
  Ref_p1/1 -> Sum/1
  Demux/2 -> Sum1/1
  Ref_v1/1 -> Sum1/2
  PID Controller/1 -> Demux1/1
  Demux1/2 -> Add/2
  Add/1 -> u07/1
  Demux1/1 -> Add/1
  Mux/1 -> PID Controller/1
  Sum1/1 -> Mux/2
  Sum/1 -> Mux/1

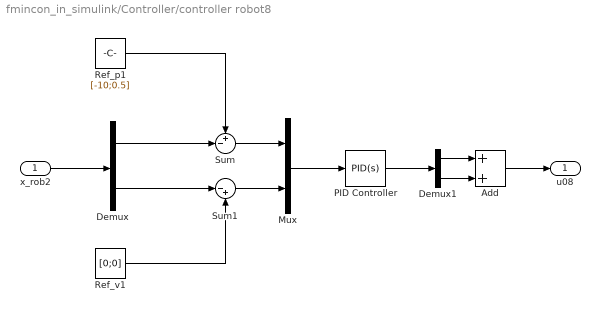
== system fmincon_in_simulink/Controller/controller robot8 ==
  x_rob2 : Inport
  Add : Sum
  Demux : Demux  Outputs=2
  Demux1 : Demux  Outputs=2
  Mux : Mux  Inputs=2
  PID Controller : slpidlib/PID Controller  Controller=PID  Form=Parallel  TimeDomain=Continuous-time  UseExternalTs=off  SampleTime=-1  IntegratorMethod=Forward Euler  FilterMethod=Forward Euler  ControllerParametersSource=internal  P=5  I=0  UseKiTs=off  D=0  N=100  UseFilter=on  TunerSelectOption=Transfer Function Based (PID Tuner App)  InitialConditionSource=internal  InitialConditionForIntegrator=0  InitialConditionForFilter=0  DifferentiatorICPrevScaledInput=0  ExternalReset=none  TrackingMode=off  Kt=1  LimitOutput=off  SatLimitsSource=internal  UpperSaturationLimit=inf  LowerSaturationLimit=-inf  LinearizeAsGain=on  AntiWindupMode=none  Kb=1  POutMin=[]  POutMax=[]  IOutMin=[]  IOutMax=[]  DOutMin=[]  DOutMax=[]  NOutMin=[]  NOutMax=[]  SumOutMin=[]  SumOutMax=[]  SaturationOutMin=[]  SaturationOutMax=[]  PParamMin=[]  PParamMax=[]  IParamMin=[]  IParamMax=[]  DParamMin=[]  DParamMax=[]  NParamMin=[]  NParamMax=[]  KbParamMin=[]  KbParamMax=[]  KtParamMin=[]  KtParamMax=[]  KbOutMin=[]  KbOutMax=[]  KtOutMin=[]  KtOutMax=[]  IntegratorOutMin=[]  IntegratorOutMax=[]  FilterOutMin=[]  FilterOutMax=[]  SumI1OutMin=[]  SumI1OutMax=[]  SumI2OutMin=[]  SumI2OutMax=[]  SumI3OutMin=[]  SumI3OutMax=[]  SumI4OutMin=[]  SumI4OutMax=[]  SumDOutMin=[]  SumDOutMax=[]  DifferentiatorOutMin=[]  DifferentiatorOutMax=[]  FilterDiffOutCoefMin=[]  FilterDiffOutCoefMax=[]  ReciprocalOutMin=[]  ReciprocalOutMax=[]  SumDenOutMin=[]  SumDenOutMax=[]  SumNumOutMin=[]  SumNumOutMax=[]  DivideOutMin=[]  DivideOutMax=[]  UdiffTsProdOutMin=[]  UdiffTsProdOutMax=[]  NTsProdOutMin=[]  NTsProdOutMax=[]  UintegralTsProdOutMin=[]  UintegralTsProdOutMax=[]  UngainTsProdOutMin=[]  UngainTsProdOutMax=[]  IntegratorContinuousStateAttributes=''  IntegratorStateMustResolveToSignalObject=off  IntegratorRTWStateStorageClass=Auto  FilterContinuousStateAttributes=''  FilterStateMustResolveToSignalObject=off  FilterRTWStateStorageClass=Auto  ParallelPVariant=InternalParameters  IdealPVariant=Disabled  IVariant=InternalParameters  DVariant=InternalParameters  IntegratorVariant=Continuous  SatVariant=Disabled  AWVariant=Passthrough  PCopyVariant=Disabled  TRVariant=Disabled  FdbkBlocksVariant=Forward  IdealPFdbkVariant=Disabled  SatFdbkVariant=Disabled  DerivativeFilterVariant=ContFilter  NVariant=InternalParameters  NCopyVariant=Disabled  FilterICVariant=InternalICsFilter  IntegratorICVariant=InternalICs  ExternalResetVariant=Disabled  TRSumVariant=Passthrough  SumFdbkVariant=Disabled  SumVariant=Sum_PID  TsampFilterVariant=InternalTs  TsampNgainVariant=Passthrough  TsampIntegralVariant=Passthrough  ExternalSaturationOutDataTypeStr=Inherit: Same as second input  aMode=0
  Ref_p1 : Constant  Value=[-10;0.5]  VectorParams1D=off
  Ref_v1 : Constant  Value=[0;0]  VectorParams1D=off
  Sum : Sum  Inputs=+-|
  Sum1 : Sum  Inputs=|-+
  u08 : Outport
  wires:
  x_rob2/1 -> Demux/1
  Demux/1 -> Sum/2
  Ref_p1/1 -> Sum/1
  Demux/2 -> Sum1/1
  Ref_v1/1 -> Sum1/2
  PID Controller/1 -> Demux1/1
  Demux1/2 -> Add/2
  Add/1 -> u08/1
  Demux1/1 -> Add/1
  Mux/1 -> PID Controller/1
  Sum1/1 -> Mux/2
  Sum/1 -> Mux/1

== system fmincon_in_simulink/Robots/Robot1 ==
  In1 : Inport
  Demux : Demux  Outputs=2
  Integrator : Integrator  InitialConditionSource=external  LimitOutput=on  UpperSaturationLimit=2  LowerSaturationLimit=-2
  Integrator1 : Integrator  InitialConditionSource=external
  initial conditions : Constant  Value=[0;0;-10;0]  VectorParams1D=off
  p1 : Outport
  v1 : Outport  Port=2
  wires:
  initial conditions/1 -> Demux/1
  In1/1 -> Integrator/1  "u1"
  Demux/1 -> Integrator/2  "v0"
  Integrator/1 -> Integrator1/1, v1/1  "v"
  Demux/2 -> Integrator1/2  "p0"
  Integrator1/1 -> p1/1  "p"

== system fmincon_in_simulink/Robots/Robot2 ==
  In1 : Inport
  Demux : Demux  Outputs=2
  Integrator : Integrator  InitialConditionSource=external  LimitOutput=on  UpperSaturationLimit=2  LowerSaturationLimit=-2
  Integrator1 : Integrator  InitialConditionSource=external
  initial conditions : Constant  Value=[0;0;-10;-10]  VectorParams1D=off
  p2 : Outport
  v2 : Outport  Port=2
  wires:
  initial conditions/1 -> Demux/1
  In1/1 -> Integrator/1  "u1"
  Demux/1 -> Integrator/2  "v0"
  Integrator/1 -> v2/1, Integrator1/1  "v"
  Demux/2 -> Integrator1/2  "p0"
  Integrator1/1 -> p2/1  "p"

== system fmincon_in_simulink/Robots/Robot3 ==
  In1 : Inport
  Demux : Demux  Outputs=2
  Integrator : Integrator  InitialConditionSource=external  LimitOutput=on  UpperSaturationLimit=2  LowerSaturationLimit=-2
  Integrator1 : Integrator  InitialConditionSource=external
  initial conditions : Constant  Value=[0;0;-10;10]  VectorParams1D=off
  p3 : Outport
  v3 : Outport  Port=2
  wires:
  initial conditions/1 -> Demux/1
  In1/1 -> Integrator/1  "u1"
  Demux/1 -> Integrator/2  "v0"
  Integrator/1 -> v3/1, Integrator1/1  "v"
  Demux/2 -> Integrator1/2  "p0"
  Integrator1/1 -> p3/1  "p"

== system fmincon_in_simulink/Robots/Robot4 ==
  In1 : Inport
  Demux : Demux  Outputs=2
  Integrator : Integrator  InitialConditionSource=external  LimitOutput=on  UpperSaturationLimit=2  LowerSaturationLimit=-2
  Integrator1 : Integrator  InitialConditionSource=external
  initial conditions : Constant  Value=[0;0;0;10]  VectorParams1D=off
  p4 : Outport
  v4 : Outport  Port=2
  wires:
  initial conditions/1 -> Demux/1
  In1/1 -> Integrator/1  "u1"
  Demux/1 -> Integrator/2  "v0"
  Integrator/1 -> v4/1, Integrator1/1  "v"
  Demux/2 -> Integrator1/2  "p0"
  Integrator1/1 -> p4/1  "p"

== system fmincon_in_simulink/Robots/Robot5 ==
  In1 : Inport
  Demux : Demux  Outputs=2
  Integrator : Integrator  InitialConditionSource=external  LimitOutput=on  UpperSaturationLimit=2  LowerSaturationLimit=-2
  Integrator1 : Integrator  InitialConditionSource=external
  initial conditions : Constant  Value=[0;0;-1;-10]  VectorParams1D=off
  p5 : Outport
  v5 : Outport  Port=2
  wires:
  initial conditions/1 -> Demux/1
  In1/1 -> Integrator/1  "u1"
  Demux/1 -> Integrator/2  "v0"
  Integrator/1 -> v5/1, Integrator1/1  "v"
  Demux/2 -> Integrator1/2  "p0"
  Integrator1/1 -> p5/1  "p"

== system fmincon_in_simulink/Robots/Robot6 ==
  In1 : Inport
  Demux : Demux  Outputs=2
  Integrator : Integrator  InitialConditionSource=external  LimitOutput=on  UpperSaturationLimit=2  LowerSaturationLimit=-2
  Integrator1 : Integrator  InitialConditionSource=external
  initial conditions : Constant  Value=[0;0;8;8]  VectorParams1D=off
  p6 : Outport
  v6 : Outport  Port=2
  wires:
  initial conditions/1 -> Demux/1
  In1/1 -> Integrator/1  "u1"
  Demux/1 -> Integrator/2  "v0"
  Integrator/1 -> v6/1, Integrator1/1  "v"
  Demux/2 -> Integrator1/2  "p0"
  Integrator1/1 -> p6/1  "p"

== system fmincon_in_simulink/Robots/Robot7 ==
  In1 : Inport
  Demux : Demux  Outputs=2
  Integrator : Integrator  InitialConditionSource=external  LimitOutput=on  UpperSaturationLimit=2  LowerSaturationLimit=-2
  Integrator1 : Integrator  InitialConditionSource=external
  initial conditions : Constant  Value=[0;0;10;-10]  VectorParams1D=off
  p7 : Outport
  v7 : Outport  Port=2
  wires:
  initial conditions/1 -> Demux/1
  In1/1 -> Integrator/1  "u1"
  Demux/1 -> Integrator/2  "v0"
  Integrator/1 -> v7/1, Integrator1/1  "v"
  Demux/2 -> Integrator1/2  "p0"
  Integrator1/1 -> p7/1  "p"

== system fmincon_in_simulink/Robots/Robot8 ==
  In1 : Inport
  Demux : Demux  Outputs=2
  Integrator : Integrator  InitialConditionSource=external  LimitOutput=on  UpperSaturationLimit=2  LowerSaturationLimit=-2
  Integrator1 : Integrator  InitialConditionSource=external
  initial conditions : Constant  Value=[0;0;12;-3]  VectorParams1D=off
  p8 : Outport
  v8 : Outport  Port=2
  wires:
  initial conditions/1 -> Demux/1
  In1/1 -> Integrator/1  "u1"
  Demux/1 -> Integrator/2  "v0"
  Integrator/1 -> v8/1, Integrator1/1  "v"
  Demux/2 -> Integrator1/2  "p0"
  Integrator1/1 -> p8/1  "p"

== system fmincon_in_simulink/Robots/Visualization ==
  p : Inport
  MATLAB Function : MATLAB Function  TreatAsAtomicUnit=on
  wires:
  p/1 -> MATLAB Function/1(p)

== matlab function fmincon_in_simulink/Controller CLF-CBF QP/MATLAB Function2 ==
  data: u0 input double; fx input; a1 output; gx input; vx input; dvx input; hx input; dhx input; u_max input; u_min input; H input; p input; a2 output; b1 output; b2 output
function [a1, a2, b1, b2] = fcn(u0, fx, gx, vx, dvx, hx, dhx, u_max, u_min, H, p)
% Dimensions
E=28;
m=16;

% Alpha(h(x)) --> class K extended
alpha1 = 0.5;
alpha2 = 3;

alpha = -alpha1*(hx.^alpha2);

% Gamma(V(x)) --> class K
gamma1 = 0.5;
gamma2 = 3;

gamma = gamma1*(vx.^gamma2);

%% QP PROBLEM
% Define FMINCON options
options = optimoptions(@fmincon, 'Algorithm','sqp');

% Define QP objective function
obj = @(x) x(1:m).' * H * x(1:m) + p*x(m+1);

% Define initial conditions
x0 = double(zeros(1,m+1));

% Define nonlinear constraints coefficients

a1 = dvx*fx + gamma;      % LfV + gamma(V)
a2 = dvx*gx;              % LgV
b1 = -dhx*fx - alpha;     % -Lfh - alpha(h)
b2 = -dhx*gx;             % -Lgh

% nonlcon = @mycon(x) [a1 + a2*x(1:16) - x(17);
%                      b1 + b2*x(1:16);
%                      []];
% 
% q1 = @getq1(x) a1 + a2*x(1:16) - x(17);
% q2 = @getq2(x) b1 + b2*x(1:16);
% qe = []


% nonlcon = @mycon;

u_opt = fmincon(obj, x0, [], [], [], [], u_min, u_max, nonlcon, options);
% u_opt = 1;

== matlab function fmincon_in_simulink/Controller/Signal Routing ==
  data: states input; x_rob1 output; x_rob2 output; x_rob3 output; x_rob4 output; x_rob5 output; x_rob6 output; x_rob7 output; x_rob8 output
function [x_rob1, x_rob2, x_rob3, x_rob4, x_rob5, x_rob6, x_rob7, x_rob8] = fcn(states)


x_rob1 = [states(1); states(2); states(17); states(18)];
x_rob2 = [states(3); states(4); states(19); states(20)];
x_rob3 = [states(5); states(6); states(21); states(22)];
x_rob4 = [states(7); states(8); states(23); states(24)];
x_rob5 = [states(9); states(10); states(25); states(26)];
x_rob6 = [states(11); states(12); states(27); states(28)];
x_rob7 = [states(13); states(14); states(29); states(30)];
x_rob8 = [states(15); states(16); states(31); states(32)];

== matlab function fmincon_in_simulink/Robots/Signal Reshaping ==
  data: p1 input; p output; v1 input; p2 input; v2 input; p3 input; v3 input; p4 input; v4 input; p5 input; v5 input; p6 input; v6 input; p7 input; v7 input; p8 input; v8 input; v output
function [p,v] = fcn(p1,v1,p2,v2,p3,v3,p4,v4,p5,v5,p6,v6,p7,v7,p8,v8)

p = [p1;p2;p3;p4;p5;p6;p7;p8;];
v = [v1;v2;v3;v4;v5;v6;v7;v8;];

== matlab function fmincon_in_simulink/Robots/Visualization/MATLAB Function ==
  data: p input
function fcn(p)
Nrobots = 8;                    % number of robots in simulation
RobotRadius = 0.25;                % desired robot radius
colors = {"red", "blue", "green", "cyan", "magenta", "black", "yellow", "#EDB120"}; %colors

x = [p(1); p(3); p(5); p(7); p(9); p(11); p(13); p(15)];
y = [p(2); p(4); p(6); p(8); p(10); p(12); p(14); p(16)];

StartPos = [x y];




for i=1:Nrobots
    
    % create the ith robot 
    pos = [StartPos(i,:)-RobotRadius 2*RobotRadius 2*RobotRadius]; %position of the robot by considering its radius
    r = rectangle('Position', pos, 'Curvature',[1 1], 'FaceColor', colors{i}, 'Edgecolor','none'); %graph of the robot as it were a kind of circle, for simplicity
    
    axis([-20 20 -20 20]) %axis of the graph: x axis from 0 to 100, the same for y
    title('Robots simulation');
    figure(1); hold on;
    %pause(0.5); 
    
    
    

end

% clf

== matlab function fmincon_in_simulink/Controller CLF-CBF QP/dh ==
  data: states input size=32; qx output size=[28 32]
function qx = fcn(states)
p1 = states(1:2);
p2 = states(3:4);
p3 = states(5:6);
p4 = states(7:8);
p5 = states(9:10);
p6 = states(11:12);
p7 = states(13:14);
p8 = states(15:16);

v1 = states(17:18);
v2 = states(19:20);
v3 = states(21:22);
v4 = states(23:24);
v5 = states(25:26);
v6 = states(27:28);
v7 = states(29:30);
v8 = states(31:32);

qx = CBF8Robots_dh(states);

== matlab function fmincon_in_simulink/Controller CLF-CBF QP/h ==
  data: states input size=32; hx output size=28
function hx = fcn(states)

p1 = states(1:2);
p2 = states(3:4);
p3 = states(5:6);
p4 = states(7:8);
p5 = states(9:10);
p6 = states(11:12);
p7 = states(13:14);
p8 = states(15:16);

v1 = states(17:18);
v2 = states(19:20);
v3 = states(21:22);
v4 = states(23:24);
v5 = states(25:26);
v6 = states(27:28);
v7 = states(29:30);
v8 = states(31:32);

hx = CBF8Robots_h(states);

== matlab function fmincon_in_simulink/Controller CLF-CBF QP/vx ==
  data: states input; vx output
function vx = fcn(states)

p1 = states(1:2);
p2 = states(3:4);
p3 = states(5:6);
p4 = states(7:8);
p5 = states(9:10);
p6 = states(11:12);
p7 = states(13:14);
p8 = states(15:16);

v1 = states(17:18);
v2 = states(19:20);
v3 = states(21:22);
v4 = states(23:24);
v5 = states(25:26);
v6 = states(27:28);
v7 = states(29:30);
v8 = states(31:32);

vx = CBF8Robots_vx(states);

== matlab function fmincon_in_simulink/Controller CLF-CBF QP/dvx ==
  data: states input; dvx output
function dvx = fcn(states)

p1 = states(1:2);
p2 = states(3:4);
p3 = states(5:6);
p4 = states(7:8);
p5 = states(9:10);
p6 = states(11:12);
p7 = states(13:14);
p8 = states(15:16);

v1 = states(17:18);
v2 = states(19:20);
v3 = states(21:22);
v4 = states(23:24);
v5 = states(25:26);
v6 = states(27:28);
v7 = states(29:30);
v8 = states(31:32);

dvx = CBF8Robots_dvx(states);

== matlab function fmincon_in_simulink/Controller CLF-CBF QP/MATLAB Function1 ==
  data: u0 input; fx input; u_opt output; gx input; vx input; dvx input; hx input; dhx input; u_max input; u_min input; H input; p input
function u_opt = regressor(u0, fx, gx, vx, dvx, hx, dhx, u_max, u_min, H, p)
    coder.extrinsic('opt_problem');
    u_opt = zeros(16,1);
    
    u = opt_problem(u0, fx, gx, vx, dvx, hx, dhx, u_max, u_min, H, p);
    u_opt = u(1:16);
end
